simulink model "Zadatak1_2012"  (R2016b)
settings: Solver=ode45  StartTime=0.0  StopTime=10.0  RelTol=1e-3  EnableMultiTasking=on
values from neighbouring files (symbols this model uses):
  ki = 150    [Zadatak1_konstatnte.m]
  kp = 10    [Zadatak1_konstatnte.m]
  T = 0.1    [Zadatak1_konstatnte.m]    (also in primer01_konstante.m = 1; primer06_konstante.m)
settings Model: Creator=Jelena  LastModifiedBy=User
settings DataIOCC: SaveFormat=StructureWithTime
settings OptimizationCC: LifeSpan=inf
settings DebuggingCC: FcnCallInpInsideContextMsg=warning  SFUnexpectedBacktrackingDiag=warning  SFNoUnconditionalDefaultTransitionDiag=warning  SFExecutionAtInitializationDiag=none
settings HardwareCC: ProdBitPerSizeT=32  ProdBitPerPtrDiffT=32  ProdWordSize=32  ProdHWDeviceType=Specified
settings GRTTargetCC: TargetLangStandard=C89/C90 (ANSI)  GeneratePreprocessorConditionals=Disable all
settings ConfigComp: CovMetricSettings=dw  CovHtmlReporting=on  CovSaveCumulativeToWorkspaceVar=on  CovSaveSingleToWorkspaceVar=on  CovExternalEMLEnable=off

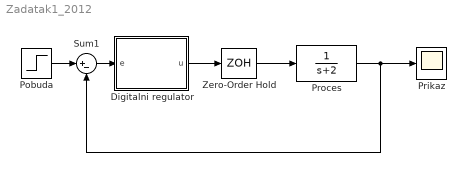
== system Zadatak1_2012 ==
  Digitalni regulator : MATLAB Function  TreatAsAtomicUnit=on
  Pobuda : Step  Time=0  SampleTime=0
  Prikaz : Scope
  Proces : TransferFcn  Denominator=[1 2]
  Sum1 : Sum  Inputs=|+-
  Zero-Order Hold : ZeroOrderHold  SampleTime=T
  wires:
  Proces/1 -> Prikaz/1, Sum1/2
  Sum1/1 -> Digitalni regulator/1(e)
  Pobuda/1 -> Sum1/1
  Zero-Order Hold/1 -> Proces/1
  Digitalni regulator/1(u) -> Zero-Order Hold/1

== matlab function Zadatak1_2012/Digitalni regulator ==
  settings: updateMethod=DISCRETE  sampleTime=T
  data: e input; u output; T parameter; ki parameter; kp parameter
function u = fcn(e, T, ki, kp)
persistent ep up;

% Inicijalizacija persistent promenljivih
if isempty(ep)
    ep = 0;
end

if isempty(up)
    up = 0;
end

% Upravljacki algoritam
u = up + (kp + ki*T)*e - kp*ep;

% Azuriranje promenljivih
up = u;
ep = e;
